simulink model "c5msim1"  (R2021b)
settings: Solver=VariableStepAuto  StartTime=0  StopTime=3  RelTol=1e-3
PreLoadFcn:
  | ww=[1e-5 1e5]; N=20;
settings Model: Creator=xuedi  LastModifiedBy=xuedi
settings DataIOCC: SaveFormat=Array  ReturnWorkspaceOutputs=off

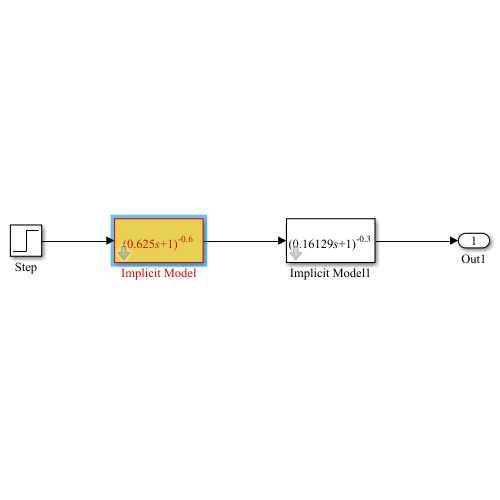
[thumbnail: Simulink's stored preview of the top-level diagram]
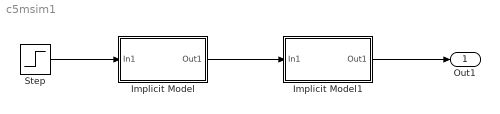
== system c5msim1 ==
  Implicit Model : Subsystem  mask{tau=1/1.6, nu=0.6, ww=ww, N=N}
      mask prompts: tau "Time constant tau"; nu "power nu"; ww "Frequency range ww"; N "Filter order"
      mask init:
      | str=['(' num2str(tau) '{\its}+1)^{' num2str(-nu) '}'];
      mask Display: disp(str,'texmode','on')
  Implicit Model1 : Subsystem  mask{tau=1/6.2, nu=0.3, ww=ww, N=N}
      mask prompts: tau "Time constant tau"; nu "power nu"; ww "Frequency range ww"; N "Filter order"
      mask init:
      | str=['(' num2str(tau) '{\its}+1)^{' num2str(-nu) '}'];
      mask Display: disp(str,'texmode','on')
  Step : Step  Time=0  SampleTime=0
  Out1 : Outport
  wires:
  Step/1 -> Implicit Model/1(In1)
  Implicit Model/1(Out1) -> Implicit Model1/1(In1)
  Implicit Model1/1(Out1) -> Out1/1

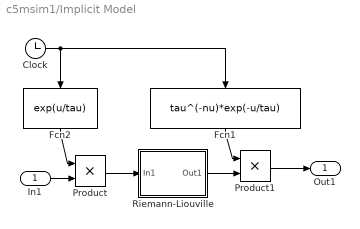
== system c5msim1/Implicit Model ==
  In1 : Inport
  Clock : Clock
  Fcn1 : Fcn  Expr=tau^(-nu)*exp(-u/tau)
  Fcn2 : Fcn  Expr=exp(u/tau)
  Product : Product
  Product1 : Product
  "Riemann-Liouville " : Subsystem  mask{gam=-nu, ww=ww, n=N, kF1=on, kF=Oustaloup filter}
      mask prompts: gam "Derivative order gamma"; ww "Frequency range [wb,wh]"; n "Apprixmation order"; kF1 "Is a low-pass filter required?"; kF "Filter type"
      mask init:
      | wb=ww(1); wh=ww(2); 
      | if kF==1, G=ousta_fod(gam,n,wb,wh);
      | else, G=new_fod(gam,n,wb,wh); end
      | G=tf(G); num=G.num{1}; den=G.den{1}; T=1/wh; 
      | if isnumeric(gam), str=['{\its}^{' num2str(gam) '}']; 
      | else, str='{\its}^{gam}'; end
      | if kF1==1, G=G*tf(1,[T 1]); end
      mask TypeOptions kF: Oustaloup filter | Modified Oustaloup filter | Matsuda-Fujii filter
      mask Display: disp(str,'texmode','on')
  Out1 : Outport
  wires:
  Product1/1 -> Out1/1
  In1/1 -> Product/2
  Fcn2/1 -> Product/1
  Product/1 -> "Riemann-Liouville "/1(In1)
  "Riemann-Liouville "/1(Out1) -> Product1/2
  Fcn1/1 -> Product1/1
  Clock/1 -> Fcn2/1, Fcn1/1

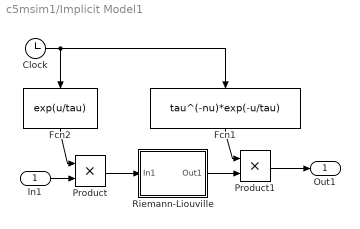
== system c5msim1/Implicit Model1 ==
  In1 : Inport
  Clock : Clock
  Fcn1 : Fcn  Expr=tau^(-nu)*exp(-u/tau)
  Fcn2 : Fcn  Expr=exp(u/tau)
  Product : Product
  Product1 : Product
  "Riemann-Liouville " : Subsystem  mask{gam=-nu, ww=ww, n=N, kF1=on, kF=Oustaloup filter}
      mask prompts: gam "Derivative order gamma"; ww "Frequency range [wb,wh]"; n "Apprixmation order"; kF1 "Is a low-pass filter required?"; kF "Filter type"
      mask init: same as c5msim1/Implicit Model/Riemann-Liouville 
      mask TypeOptions kF: Oustaloup filter | Modified Oustaloup filter | Matsuda-Fujii filter
      mask Display: disp(str,'texmode','on')
  Out1 : Outport
  wires:
  Product1/1 -> Out1/1
  In1/1 -> Product/2
  Fcn2/1 -> Product/1
  Product/1 -> "Riemann-Liouville "/1(In1)
  "Riemann-Liouville "/1(Out1) -> Product1/2
  Fcn1/1 -> Product1/1
  Clock/1 -> Fcn2/1, Fcn1/1

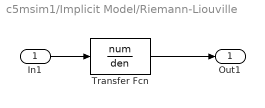
== system c5msim1/Implicit Model/Riemann-Liouville  ==
  In1 : Inport
  Transfer Fcn : TransferFcn  Numerator=num  Denominator=den
  Out1 : Outport
  wires:
  Transfer Fcn/1 -> Out1/1
  In1/1 -> Transfer Fcn/1

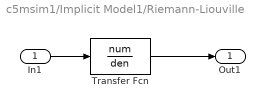
== system c5msim1/Implicit Model1/Riemann-Liouville  ==
  In1 : Inport
  Transfer Fcn : TransferFcn  Numerator=num  Denominator=den
  Out1 : Outport
  wires:
  Transfer Fcn/1 -> Out1/1
  In1/1 -> Transfer Fcn/1
